simulink model "CSE1_CV3_1Straight"  (Simulink 7.3)
settings: Solver=ode4  StartTime=0.0  StopTime=inf  FixedStep=0.1  RelTol=1e-3
undefined symbols (not defined in the file or in its folder): eta1_0_real, v1_0_real, velocitySatValues1
libraries: simulink x68, dspmtrx3 x24, simulink_extras x23, marine_gnc x5, dspindex x5, dspinverses x4
(part 1 of 6)
settings Model: Creator=Dinh  LastModifiedBy=mcl  BufferReuse=off
settings DataIOCC: LimitDataPoints=off  SaveOutput=off  SaveTime=off
settings OptimizationCC: BlockReduction=off  BooleanDataType=off  ConditionallyExecuteInputs=off  OptimizeBlockIOStorage=off  BufferReuse=off  ExpressionFolding=off  LocalBlockOutputs=off  SimCompilerOptimization=On
settings DebuggingCC: InheritedTsInSrcMsg=none
settings SFSimCC: SimBuildMode=sf_nonincremental_build
settings RTWCC: SystemTargetFile=nidll.tlc  TemplateMakefile=nidll_vc.tmf  Description=NI Real-Time Target for Release 2007b or later  ProcessScript=nidll_make_rtw_hook
settings STFCustomTargetCC: MatFileLogging=on  SystemTargetFile=nidll.tlc

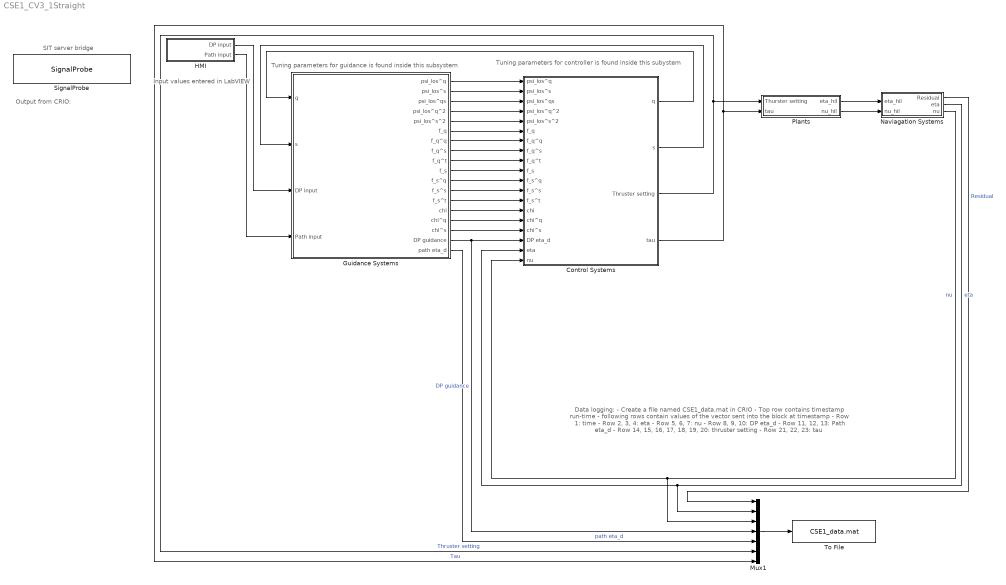
== system CSE1_CV3_1Straight ==
  note: Output from CRIO:
  note: SIT server bridge
  note: Tuning parameters for controller is found inside this subystem
  note: Tuning parameters for guidance is found inside this subsystem
  note: Input values entered
      |  in LabVIEW
  note: Data logging:
      | - Create a file named CSE1_data.mat in CRIO
      | - Top row contains timestamp run-time
      | - following rows contain values of the vector sent into the block at timestamp
      | - Row 1: time
      | - Row 2, 3, 4: eta
      | - Row 5, 6, 7: nu
      | - Row 8, 9, 10: DP eta_d
      | - Row 11, 12, 13: Path eta_d
      | - Row 14, 15, 16, 17, 18, 19, 20: thruster setting
      | - Row 21, 22, 23: tau
  Control Systems : Subsystem
  Guidance Systems : Subsystem
  HMI : Subsystem
  Mux1 : Mux  Inputs=7
  Naviagation Systems : Subsystem
      settings: MinAlgLoopOccurrences=on
  Plants : Subsystem
  SignalProbe : S-Function  Description=Use this block with SIT.  FunctionName=SignalProbe  Parameters=1  EnableBusSupport=off
      settings: PreSaveFcn=NISIT_ModelVars;
      mask Description: The LabVIEW Simulation Interface Toolkit uses the SignalProbe block to probe the signals in the model. The SignalProbe block must be on the top level of the model hierarchy. You can have only one SignalProbe block per model file. Do not rename the SignalProbe block. Do not change the name of another model block to SignalProbe.
  To File : ToFile  Filename=CSE1_data.mat  MatrixName=cse1_data
  wires:
  Control Systems/3(Thruster setting) -> Plants/1(Thurster setting), Mux1/6  "Thruster setting"
  Guidance Systems/17(DP guidance) -> Control Systems/17(DP eta_d), Mux1/4  "DP guidance"
  Plants/1(eta_hil) -> Naviagation Systems/1(eta_hil)
  Plants/2(nu_hil) -> Naviagation Systems/2(nu_hil)
  Naviagation Systems/2(eta) -> Mux1/2, Control Systems/18(eta)  "eta"
  Naviagation Systems/3(nu) -> Control Systems/19(nu), Mux1/3  "nu"
  Mux1/1 -> To File/1
  HMI/1(DP input) -> Guidance Systems/3(DP input)
  Control Systems/1(q) -> Guidance Systems/1(q)
  Control Systems/2(s) -> Guidance Systems/2(s)
  Control Systems/4(tau) -> Plants/2(tau), Mux1/7  "Tau"
  Naviagation Systems/1(Residual) -> Mux1/1  "Residual"
  HMI/2(Path input) -> Guidance Systems/4(Path input)
  Guidance Systems/18(path eta_d) -> Mux1/5  "path eta_d"
  Guidance Systems/1(psi_los^q) -> Control Systems/1(psi_los^q)
  Guidance Systems/2(psi_los^s) -> Control Systems/2(psi_los^s)
  Guidance Systems/3(psi_los^qs) -> Control Systems/3(psi_los^qs)
  Guidance Systems/4(psi_los^q^2) -> Control Systems/4(psi_los^q^2)
  Guidance Systems/5(psi_los^s^2) -> Control Systems/5(psi_los^s^2)
  Guidance Systems/6(f_q) -> Control Systems/6(f_q)
  Guidance Systems/7("f_q^q ") -> Control Systems/7(f_q^q)
  Guidance Systems/8(f_q^s) -> Control Systems/8(f_q^s)
  Guidance Systems/9(f_q^t) -> Control Systems/9(f_q^t)
  Guidance Systems/10(f_s) -> Control Systems/10(f_s)
  Guidance Systems/11(f_s^q) -> Control Systems/11(f_s^q)
  Guidance Systems/12(f_s^s) -> Control Systems/12(f_s^s)
  Guidance Systems/13(f_s^t) -> Control Systems/13(f_s^t)
  Guidance Systems/15(chi^q) -> Control Systems/15(chi^q)
  Guidance Systems/16(chi^s) -> Control Systems/16(chi^s)
  Guidance Systems/14(chi) -> Control Systems/14(chi)

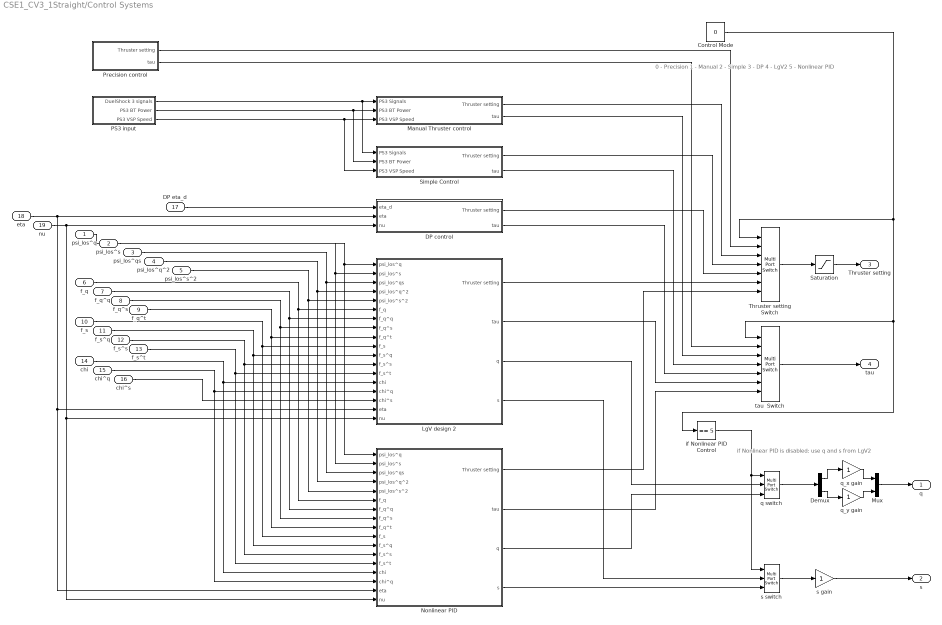
== system CSE1_CV3_1Straight/Control Systems ==
  note: 0 - Precision
      | 1 - Manual
      | 2 - Simple
      | 3 - DP
      | 4 - LgV2
      | 5 - Nonlinear PID
  note: if Nonlinear PID is disabled:
      |  use q and s from LgV2
  psi_los^q : Inport
  psi_los^s : Inport  Port=2
  psi_los^qs : Inport  Port=3
  psi_los^q^2 : Inport  Port=4
  psi_los^s^2 : Inport  Port=5
  f_q : Inport  Port=6
  f_q^q : Inport  Port=7
  f_q^s : Inport  Port=8
  f_q^t : Inport  Port=9
  f_s : Inport  Port=10
  f_s^q : Inport  Port=11
  f_s^s : Inport  Port=12
  f_s^t : Inport  Port=13
  chi : Inport  Port=14
  chi^q : Inport  Port=15
  chi^s : Inport  Port=16
  DP eta_d : Inport  Port=17
  eta : Inport  Port=18
  nu : Inport  Port=19
  Control Mode : Constant  Value=0
  DP control : Subsystem
  Demux : Demux  Outputs=2
  LgV design 2 : Subsystem
  Manual Thruster control : Subsystem
      settings: MinAlgLoopOccurrences=on
  Mux : Mux  Inputs=2
  Nonlinear PID : Subsystem
  PS3 input : Subsystem
  Precision control : Subsystem
  Saturation : Saturate  UpperLimit=1.0  LowerLimit=-1.0
  Simple Control : Subsystem
      settings: MinAlgLoopOccurrences=on
  Thruster setting Switch : MultiPortSwitch  Inputs=6  zeroidx=on
  if Nonlinear PID Control : simulink/Logic and Bit Operations/Compare To Constant  SystemSampleTime=-1  relop===  const=5  LogicOutDataTypeMode=uint8
  q switch : MultiPortSwitch  Inputs=2  zeroidx=on
  q_x gain : Gain  ParameterDataType=fixdt(1, 16)  ParameterScaling=2^0  OutDataType=fixdt(1, 16)  OutScaling=2^0
  q_y gain : Gain  ParameterDataType=fixdt(1, 16)  ParameterScaling=2^0  OutDataType=fixdt(1, 16)  OutScaling=2^0
  s gain : Gain  ParameterDataType=fixdt(1, 16)  ParameterScaling=2^0  OutDataType=fixdt(1, 16)  OutScaling=2^0
  s switch : MultiPortSwitch  Inputs=2  zeroidx=on
  tau  Switch : MultiPortSwitch  Inputs=6  zeroidx=on
  q : Outport
  s : Outport  Port=2
  Thruster setting : Outport  Port=3  PortDimensions=7
  tau : Outport  Port=4
  wires:
  DP eta_d/1 -> DP control/1(eta_d)
  nu/1 -> DP control/3(nu), LgV design 2/18(nu), Nonlinear PID/17(nu)
  eta/1 -> DP control/2(eta), LgV design 2/17(eta), Nonlinear PID/16(eta)
  Control Mode/1 -> Thruster setting Switch/1, tau  Switch/1, if Nonlinear PID Control/1
  Thruster setting Switch/1 -> Saturation/1
  Saturation/1 -> Thruster setting/1
  PS3 input/1(DuelShock 3 signals) -> Manual Thruster control/1(PS3 Signals), Simple Control/1(PS3 Signals)
  PS3 input/2(PS3 BT Power) -> Manual Thruster control/2(PS3 BT Power), Simple Control/2(PS3 BT Power)
  PS3 input/3(PS3 VSP Speed) -> Manual Thruster control/3(PS3 VSP Speed), Simple Control/3(PS3 VSP Speed)
  q switch/1 -> Demux/1
  s switch/1 -> s gain/1
  tau  Switch/1 -> tau/1
  Precision control/1(Thruster setting) -> Thruster setting Switch/2
  Nonlinear PID/4(s) -> s switch/3
  Manual Thruster control/1(Thruster setting) -> Thruster setting Switch/3
  Simple Control/1(Thruster setting) -> Thruster setting Switch/4
  DP control/1(Thruster setting) -> Thruster setting Switch/5
  LgV design 2/1(Thruster setting) -> Thruster setting Switch/6
  Precision control/2(tau) -> tau  Switch/2
  Manual Thruster control/2(tau) -> tau  Switch/3
  Simple Control/2(tau) -> tau  Switch/4
  DP control/2(tau) -> tau  Switch/5
  LgV design 2/2(tau) -> tau  Switch/6
  Nonlinear PID/1(Thruster setting) -> Thruster setting Switch/7
  Nonlinear PID/2(tau) -> tau  Switch/7
  LgV design 2/3(q) -> q switch/2
  Nonlinear PID/3(q) -> q switch/3
  if Nonlinear PID Control/1 -> s switch/1, q switch/1
  psi_los^q/1 -> LgV design 2/1(psi_los^q), Nonlinear PID/1(psi_los^q)
  psi_los^s/1 -> LgV design 2/2(psi_los^s), Nonlinear PID/2(psi_los^s)
  psi_los^qs/1 -> LgV design 2/3(psi_los^qs), Nonlinear PID/3(psi_los^qs)
  psi_los^q^2/1 -> LgV design 2/4(psi_los^q^2), Nonlinear PID/4(psi_los^q^2)
  psi_los^s^2/1 -> LgV design 2/5(psi_los^s^2), Nonlinear PID/5(psi_los^s^2)
  f_q/1 -> LgV design 2/6(f_q), Nonlinear PID/6(f_q)
  f_q^q/1 -> LgV design 2/7(f_q^q), Nonlinear PID/7(f_q^q)
  f_q^s/1 -> LgV design 2/8(f_q^s), Nonlinear PID/8(f_q^s)
  f_q^t/1 -> LgV design 2/9(f_q^t), Nonlinear PID/9(f_q^t)
  f_s/1 -> LgV design 2/10(f_s), Nonlinear PID/10(f_s)
  f_s^q/1 -> LgV design 2/11(f_s^q), Nonlinear PID/11(f_s^q)
  f_s^s/1 -> LgV design 2/12(f_s^s), Nonlinear PID/12(f_s^s)
  f_s^t/1 -> LgV design 2/13(f_s^t), Nonlinear PID/13(f_s^t)
  chi/1 -> LgV design 2/14(chi), Nonlinear PID/14(chi)
  chi^q/1 -> LgV design 2/15(chi^q), Nonlinear PID/15(chi^q)
  chi^s/1 -> LgV design 2/16(chi^s)
  s gain/1 -> s/1
  Demux/1 -> q_x gain/1
  Demux/2 -> q_y gain/1
  q_x gain/1 -> Mux/1
  q_y gain/1 -> Mux/2
  Mux/1 -> q/1
  LgV design 2/4(s) -> s switch/2

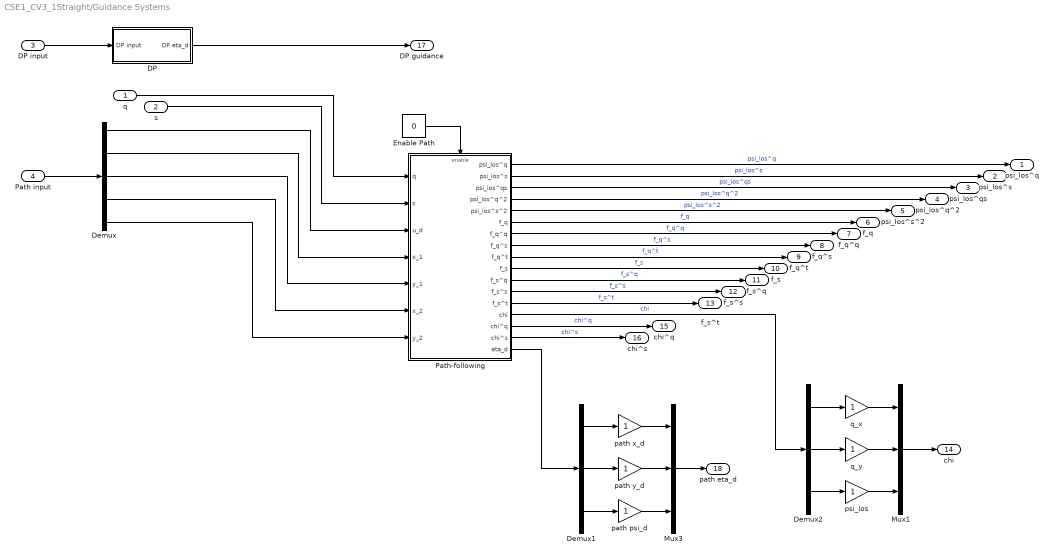
== system CSE1_CV3_1Straight/Guidance Systems ==
  q : Inport
  s : Inport  Port=2
  DP input : Inport  Port=3
  Path input : Inport  Port=4
  DP : Subsystem
  Demux : Demux  Outputs=5
  Demux1 : Demux  Outputs=3
  Demux2 : Demux  Outputs=3
  Enable Path : Constant  Value=0
  Mux1 : Mux  Inputs=3
  Mux3 : Mux  Inputs=3
  Path-following : Subsystem
  path psi_d : Gain  ParameterDataType=fixdt(1, 16)  ParameterScaling=2^0  OutDataType=fixdt(1, 16)  OutScaling=2^0
  path x_d : Gain  ParameterDataType=fixdt(1, 16)  ParameterScaling=2^0  OutDataType=fixdt(1, 16)  OutScaling=2^0
  path y_d : Gain  ParameterDataType=fixdt(1, 16)  ParameterScaling=2^0  OutDataType=fixdt(1, 16)  OutScaling=2^0
  psi_los : Gain  ParameterDataType=fixdt(1, 16)  ParameterScaling=2^0  OutDataType=fixdt(1, 16)  OutScaling=2^0
  q_x : Gain  ParameterDataType=fixdt(1, 16)  ParameterScaling=2^0  OutDataType=fixdt(1, 16)  OutScaling=2^0
  q_y : Gain  ParameterDataType=fixdt(1, 16)  ParameterScaling=2^0  OutDataType=fixdt(1, 16)  OutScaling=2^0
  psi_los^q : Outport
  psi_los^s : Outport  Port=2
  psi_los^qs : Outport  Port=3
  psi_los^q^2 : Outport  Port=4
  psi_los^s^2 : Outport  Port=5
  f_q : Outport  Port=6
  "f_q^q " : Outport  Port=7
  f_q^s : Outport  Port=8
  f_q^t : Outport  Port=9
  f_s : Outport  Port=10
  f_s^q : Outport  Port=11
  f_s^s : Outport  Port=12
  f_s^t : Outport  Port=13
  chi : Outport  Port=14
  chi^q : Outport  Port=15
  chi^s : Outport  Port=16
  DP guidance : Outport  Port=17
  path eta_d : Outport  Port=18
  wires:
  DP/1(DP eta_d) -> DP guidance/1
  DP input/1 -> DP/1(DP input)
  q/1 -> Path-following/1(q)
  s/1 -> Path-following/2(s)
  Demux/1 -> Path-following/3(u_d)
  Demux/2 -> Path-following/4(x_1)
  Demux/3 -> Path-following/5(y_1)
  Demux/4 -> Path-following/6(x_2)
  Path-following/1(psi_los^q) -> psi_los^q/1  "psi_los^q"
  Path-following/2(psi_los^s) -> psi_los^s/1  "psi_los^s"
  Path-following/3(psi_los^qs) -> psi_los^qs/1  "psi_los^qs"
  Path-following/4(psi_los^q^2) -> psi_los^q^2/1  "psi_los^q^2"
  Path-following/5(psi_los^s^2) -> psi_los^s^2/1  "psi_los^s^2"
  Path-following/6(f_q) -> f_q/1  "f_q"
  Path-following/7("f_q^q ") -> "f_q^q "/1  "f_q^q"
  Path-following/8(f_q^s) -> f_q^s/1  "f_q^s"
  Path-following/9(f_q^t) -> f_q^t/1  "f_q^t"
  Path-following/10(f_s) -> f_s/1  "f_s"
  Path-following/11(f_s^q) -> f_s^q/1  "f_s^q"
  Path-following/12(f_s^s) -> f_s^s/1  "f_s^s"
  Path-following/13(f_s^t) -> f_s^t/1  "f_s^t"
  Path-following/14(chi) -> Demux2/1  "chi"
  Path-following/15(chi^q) -> chi^q/1  "chi^q"
  Path-following/16(chi^s) -> chi^s/1  "chi^s"
  Path input/1 -> Demux/1
  Demux/5 -> Path-following/7(y_2)
  Demux1/1 -> path x_d/1
  Demux1/2 -> path y_d/1
  Demux1/3 -> path psi_d/1
  path x_d/1 -> Mux3/1
  path psi_d/1 -> Mux3/3
  path y_d/1 -> Mux3/2
  Mux3/1 -> path eta_d/1
  Path-following/17(eta_d) -> Demux1/1
  Demux2/1 -> q_x/1
  Demux2/2 -> q_y/1
  Demux2/3 -> psi_los/1
  q_x/1 -> Mux1/1
  psi_los/1 -> Mux1/3
  q_y/1 -> Mux1/2
  Mux1/1 -> chi/1
  Enable Path/1 -> Path-following/Enable

== system CSE1_CV3_1Straight/HMI ==
  DP Input : Subsystem
  Path-following input : Subsystem
  DP input : Outport
  Path input : Outport  Port=2
  wires:
  DP Input/1(DP input) -> DP input/1
  Path-following input/1(Path input) -> Path input/1

== system CSE1_CV3_1Straight/Naviagation Systems ==
  eta_hil : Inport
  nu_hil : Inport  Port=2
  Controller Input Selector : Constant  Value=0
  Demux : Demux  Outputs=3
  Demux1 : Demux  Outputs=3
  Eta Switch : MultiPortSwitch  Inputs=2  zeroidx=on
  Mux1 : Mux  Inputs=3
  Mux3 : Mux  Inputs=3
  Nu Switch : MultiPortSwitch  Inputs=2  zeroidx=on
  Qualisys 6 DOF : Subsystem
  eta_surge : Gain  ParameterDataType=fixdt(1, 16)  ParameterScaling=2^0  OutDataType=fixdt(1, 16)  OutScaling=2^0
  eta_sway : Gain  ParameterDataType=fixdt(1, 16)  ParameterScaling=2^0  OutDataType=fixdt(1, 16)  OutScaling=2^0
  eta_yaw : Gain  ParameterDataType=fixdt(1, 16)  ParameterScaling=2^0  OutDataType=fixdt(1, 16)  OutScaling=2^0
  nu_surge : Gain  ParameterDataType=fixdt(1, 16)  ParameterScaling=2^0  OutDataType=fixdt(1, 16)  OutScaling=2^0
  nu_sway : Gain  ParameterDataType=fixdt(1, 16)  ParameterScaling=2^0  OutDataType=fixdt(1, 16)  OutScaling=2^0
  nu_yaw : Gain  ParameterDataType=fixdt(1, 16)  ParameterScaling=2^0  OutDataType=fixdt(1, 16)  OutScaling=2^0
  Residual : Outport
  eta : Outport  Port=2
  nu : Outport  Port=3
  wires:
  Controller Input Selector/1 -> Eta Switch/1, Nu Switch/1
  Qualisys 6 DOF/1(eta_qs) -> Eta Switch/2
  Qualisys 6 DOF/2(nu_qs) -> Nu Switch/2
  eta_hil/1 -> Eta Switch/3
  nu_hil/1 -> Nu Switch/3
  Demux/1 -> eta_surge/1
  Demux/2 -> eta_sway/1
  Demux/3 -> eta_yaw/1
  eta_surge/1 -> Mux3/1
  eta_yaw/1 -> Mux3/3
  eta_sway/1 -> Mux3/2
  Mux3/1 -> eta/1
  Demux1/1 -> nu_surge/1
  Demux1/2 -> nu_sway/1
  Demux1/3 -> nu_yaw/1
  nu_surge/1 -> Mux1/1
  nu_sway/1 -> Mux1/2
  nu_yaw/1 -> Mux1/3
  Mux1/1 -> nu/1
  Nu Switch/1 -> Demux1/1
  Eta Switch/1 -> Demux/1
  Qualisys 6 DOF/3(Residual) -> Residual/1

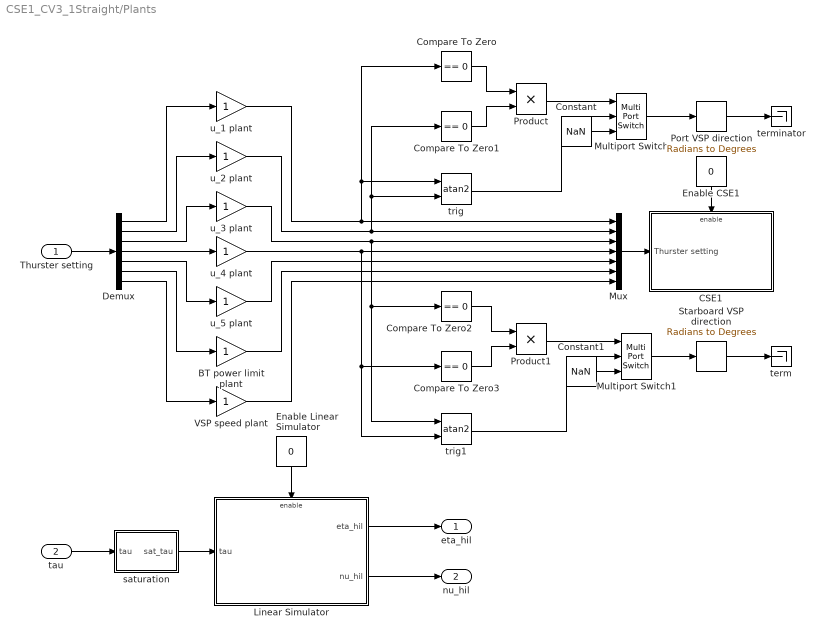
== system CSE1_CV3_1Straight/Plants ==
  Thurster setting : Inport
  tau : Inport  Port=2
  BT power limit plant : Gain  ParameterDataType=fixdt(1, 16)  ParameterScaling=2^0  OutDataType=fixdt(1, 16)  OutScaling=2^0
  CSE1 : Subsystem
  Compare To Zero{,1..3} (4 alike) : simulink/Logic and Bit Operations/Compare To Zero  SystemSampleTime=-1  relop===  LogicOutDataTypeMode=uint8  ZeroCross=off
  Constant : Constant  Value=NaN  OutDataType=fixdt(1, 16)  OutScaling=2^0
  Constant1 : Constant  Value=NaN  OutDataType=fixdt(1, 16)  OutScaling=2^0
  Demux : Demux  Outputs=7
  Enable CSE1 : Constant  Value=0
  Enable Linear Simulator : Constant  Value=0
  Linear Simulator : Subsystem
      settings: MinAlgLoopOccurrences=on
  Multiport Switch : MultiPortSwitch  Inputs=2  zeroidx=on  OutDataType=fixdt(1, 16)  OutScaling=2^0
  Multiport Switch1 : MultiPortSwitch  Inputs=2  zeroidx=on  OutDataType=fixdt(1, 16)  OutScaling=2^0
  Mux : Mux  Inputs=7
  Port VSP direction : simulink_extras/Transformations/Radians to Degrees  SystemSampleTime=-1
  Product : Product  OutDataType=fixdt(1, 16)  OutScaling=2^0  RndMeth=Zero
  Product1 : Product  OutDataType=fixdt(1, 16)  OutScaling=2^0  RndMeth=Zero
  Starboard VSP direction : simulink_extras/Transformations/Radians to Degrees  SystemSampleTime=-1
  VSP speed plant : Gain  ParameterDataType=fixdt(1, 16)  ParameterScaling=2^0  OutDataType=fixdt(1, 16)  OutScaling=2^0
  saturation : Subsystem  AncestorBlock=marine_gnc/Examples/Vessels/CyberShipII/saturation
  term : Terminator
  terminator : Terminator
  trig : Trigonometry  Operator=atan2
  trig1 : Trigonometry  Operator=atan2
  u_1 plant : Gain  ParameterDataType=fixdt(1, 16)  ParameterScaling=2^0  OutDataType=fixdt(1, 16)  OutScaling=2^0
  u_2 plant : Gain  ParameterDataType=fixdt(1, 16)  ParameterScaling=2^0  OutDataType=fixdt(1, 16)  OutScaling=2^0
  u_3 plant : Gain  ParameterDataType=fixdt(1, 16)  ParameterScaling=2^0  OutDataType=fixdt(1, 16)  OutScaling=2^0
  u_4 plant : Gain  ParameterDataType=fixdt(1, 16)  ParameterScaling=2^0  OutDataType=fixdt(1, 16)  OutScaling=2^0
  u_5 plant : Gain  ParameterDataType=fixdt(1, 16)  ParameterScaling=2^0  OutDataType=fixdt(1, 16)  OutScaling=2^0
  eta_hil : Outport
  nu_hil : Outport  Port=2
  wires:
  Linear Simulator/1(eta_hil) -> eta_hil/1
  Linear Simulator/2(nu_hil) -> nu_hil/1
  Enable CSE1/1 -> CSE1/Enable
  Enable Linear Simulator/1 -> Linear Simulator/Enable
  Thurster setting/1 -> Demux/1
  Mux/1 -> CSE1/1(Thurster setting)
  Demux/1 -> u_1 plant/1
  Demux/2 -> u_2 plant/1
  Demux/3 -> u_3 plant/1
  Demux/4 -> u_4 plant/1
  u_4 plant/1 -> Mux/4, trig1/2, Compare To Zero3/1
  u_1 plant/1 -> Mux/1, trig/1, Compare To Zero/1
  u_2 plant/1 -> Mux/2, trig/2, Compare To Zero1/1
  u_3 plant/1 -> Mux/3, trig1/1, Compare To Zero2/1
  Demux/5 -> u_5 plant/1
  Demux/6 -> BT power limit plant/1
  Demux/7 -> VSP speed plant/1
  u_5 plant/1 -> Mux/5
  BT power limit plant/1 -> Mux/6
  VSP speed plant/1 -> Mux/7
  tau/1 -> saturation/1(tau)
  saturation/1(sat_tau) -> Linear Simulator/1(tau)
  Compare To Zero/1 -> Product/1
  Compare To Zero1/1 -> Product/2
  Product/1 -> Multiport Switch/1
  Multiport Switch/1 -> Port VSP direction/1
  trig/1 -> Multiport Switch/2
  Constant/1 -> Multiport Switch/3
  Compare To Zero2/1 -> Product1/1
  Compare To Zero3/1 -> Product1/2
  Product1/1 -> Multiport Switch1/1
  Multiport Switch1/1 -> Starboard VSP direction/1
  trig1/1 -> Multiport Switch1/2
  Constant1/1 -> Multiport Switch1/3
  Port VSP direction/1 -> terminator/1
  Starboard VSP direction/1 -> term/1

== system CSE1_CV3_1Straight/Control Systems/DP control ==
  eta_d : Inport
  eta : Inport  Port=2
  nu : Inport  Port=3
  BT_power_limit : Constant  Value=0.5
  DP controller : Subsystem  mask(Nonlinear DP Controller){Kp=(0.1)^2*[25.8000 0  0;  0  33.8000  1.0115;  0  1.0115  2.7600 ], Kd=2*0.8*0.1*[25.8000 0  0;  0  33.8000  1.0115;  0  1.0115  2.7600 ], Ki=(0.1^3/10)*[25.8000 0  0;  0  33.8000  1.0115;  0  1.0115  2.7600 ]}
      mask prompts: Kp "Proportional Gain Matrix: Kp"; Kd "Derivative Gain Matrix: Kd"; Ki "Integral Gain Matrix: Ki"
      mask help: Nonlinear PID controller for Set-Point Reulation in Surge, Sway and Yaw
      mask Help:
      | The nonlinear  PID controller uses the rotation matrix in yaw for proper scaling of the surge, sway and yaw gains as a function of the yaw angle.
      | INPUTS: (1) eta_ref, (2) eta, (3) nu. OUPUTS: (1) tau.
      mask Display: disp('Nonlinear PID\n set-point controller')
  DP tau_surge : Gain  ParameterDataType=fixdt(1, 16)  ParameterScaling=2^0  OutDataType=fixdt(1, 16)  OutScaling=2^0
  DP tau_sway : Gain  ParameterDataType=fixdt(1, 16)  ParameterScaling=2^0  OutDataType=fixdt(1, 16)  OutScaling=2^0
  DP tau_yaw : Gain  ParameterDataType=fixdt(1, 16)  ParameterScaling=2^0  OutDataType=fixdt(1, 16)  OutScaling=2^0
  DP u_{1..5} (5 alike) : Gain  ParameterDataType=fixdt(1, 16)  ParameterScaling=2^0  OutDataType=fixdt(1, 16)  OutScaling=2^0
  Demux : Demux  Outputs=3
  Demux1 : Demux  Outputs=5
  Enable Filter : Constant  Value=0
  Multiport Switch : MultiPortSwitch  Inputs=2  zeroidx=on
  Multiport Switch1 : MultiPortSwitch  Inputs=2  zeroidx=on
  Mux1 : Mux  Inputs=3
  Mux2 : Mux  Inputs=5
  Mux3 : Mux  Inputs=3
  Passive DP wave filter1 : marine_gnc/Navigation/Observers/Passive DP wave filter  SystemSampleTime=-1  lambda=0.1*diag([1 1 1])  w_o=diag([0.8 0.8 0.8])  K4=0.1*diag([1 1 0.1])  K3=0.1*diag([1 1 0.1])  w_c=1.3*diag([0.8 0.8 0.8])  T_b=diag([100 100 100])  M="[ 25.8000   0    0;   0   33.8000   1.0115; 0   1.0115    2.7600 ]"  D="[2 0  0;  0 7 0.1; 0 0.1 0.5]"
  Saturation : Saturate  UpperLimit=1.0  LowerLimit=-1.0
  Thruster allocation : Subsystem
  To File : ToFile  Filename=CSE1_data_eta_w.mat  MatrixName=cse1_data
  VSP_speeds : Constant  Value=0.4
  Thruster setting : Outport  InitialOutput=[0;0;0;0;0;0;0]
  tau : Outport  Port=2
  wires:
  Mux1/1 -> Thruster setting/1
  eta_d/1 -> DP controller/1(eta_ref)
  eta/1 -> Passive DP wave filter1/1, Multiport Switch/2
  nu/1 -> Multiport Switch1/2
  Multiport Switch/1 -> DP controller/2(eta)
  Multiport Switch1/1 -> DP controller/3(nu)
  Passive DP wave filter1/2 -> Multiport Switch/3
  Passive DP wave filter1/3 -> Multiport Switch1/3
  Enable Filter/1 -> Multiport Switch/1, Multiport Switch1/1
  Saturation/1 -> Mux1/1
  Passive DP wave filter1/1 -> To File/1
  BT_power_limit/1 -> Mux1/2
  VSP_speeds/1 -> Mux1/3
  Demux/1 -> DP tau_surge/1
  Demux/2 -> DP tau_sway/1
  Demux/3 -> DP tau_yaw/1
  DP tau_surge/1 -> Mux3/1
  DP tau_yaw/1 -> Mux3/3
  DP tau_sway/1 -> Mux3/2
  DP controller/1(tau) -> Demux/1
  Mux3/1 -> Thruster allocation/1(tau), Passive DP wave filter1/2, tau/1
  Demux1/1 -> DP u_1/1
  Demux1/2 -> DP u_2/1
  Demux1/3 -> DP u_3/1
  DP u_1/1 -> Mux2/1
  DP u_3/1 -> Mux2/3
  DP u_2/1 -> Mux2/2
  Demux1/4 -> DP u_4/1
  Demux1/5 -> DP u_5/1
  DP u_4/1 -> Mux2/4
  DP u_5/1 -> Mux2/5
  Mux2/1 -> Saturation/1
  Thruster allocation/1(u_act) -> Demux1/1

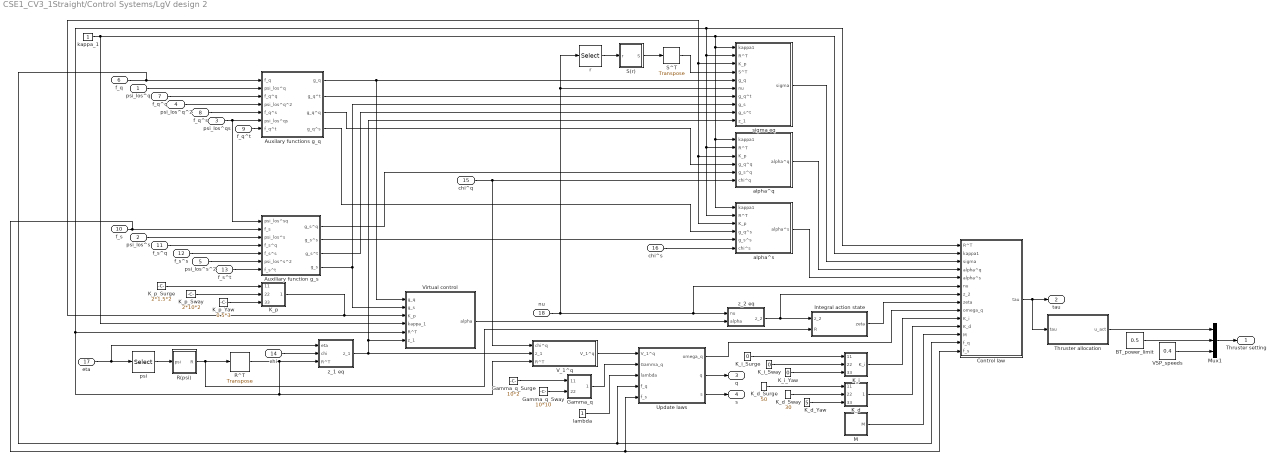
== system CSE1_CV3_1Straight/Control Systems/LgV design 2 ==
  psi_los^q : Inport
  psi_los^s : Inport  Port=2
  psi_los^qs : Inport  Port=3
  psi_los^q^2 : Inport  Port=4
  psi_los^s^2 : Inport  Port=5
  f_q : Inport  Port=6
  f_q^q : Inport  Port=7
  f_q^s : Inport  Port=8
  f_q^t : Inport  Port=9
  f_s : Inport  Port=10
  f_s^q : Inport  Port=11
  f_s^s : Inport  Port=12
  f_s^t : Inport  Port=13
  chi : Inport  Port=14
  chi^q : Inport  Port=15
  chi^s : Inport  Port=16
  eta : Inport  Port=17
  nu : Inport  Port=18
  Auxilary functions g_q : Subsystem
  Auxiliary function g_s : Subsystem
  BT_power_limit : Constant  Value=0.5
  Control law : Subsystem
  Gamma_q : Subsystem
  Gamma_q_Surge : Constant  Value=10*2
  Gamma_q_Sway : Constant  Value=10*10
  Integral action state : Subsystem
  K_d : Subsystem
  K_d_Surge : Constant  Value=50
  K_d_Sway : Constant  Value=30
  K_d_Yaw : Constant  Value=5
  K_i : Subsystem
  K_i_Surge : Constant  Value=0
  K_i_Sway : Constant  Value=0
  K_i_Yaw : Constant  Value=0
  K_p : Subsystem
  K_p_Surge : Constant  Value=2*1.5*2
  K_p_Sway : Constant  Value=2*10*2
  K_p_Yaw : Constant  Value=0.5*3
  M : Subsystem
  Mux1 : Mux  Inputs=3
  R(psi) : Subsystem
  R^T : dspmtrx3/Transpose  SystemSampleTime=-1  Hermitian=off  overflowFlag=off
  S(r) : Subsystem
  S^T : dspmtrx3/Transpose  SystemSampleTime=-1  Hermitian=off  overflowFlag=off
  Thruster allocation : Subsystem
  Update laws : Subsystem
  VSP_speeds : Constant  Value=0.4
  V_1^q : Subsystem
  Virtual control : Subsystem
  alpha^q : Subsystem
  alpha^s : Subsystem
  kappa_1 : Constant
  lambda : Constant
  psi : Selector  InputPortWidth=3  IndexOptions=Index vector (dialog)  Indices=[3]  OutputSizes=1
  r : Selector  InputPortWidth=3  IndexOptions=Index vector (dialog)  Indices=[3]  OutputSizes=1
  sigma eq : Subsystem
  z_1 eq : Subsystem
  z_2 eq : Subsystem
  Thruster setting : Outport  InitialOutput=[0;0;0;0;0;0;0]
  tau : Outport  Port=2
  q : Outport  Port=3
  s : Outport  Port=4
  wires:
  psi/1 -> R(psi)/1(psi)
  eta/1 -> psi/1, z_1 eq/1(eta)
  R(psi)/1(R) -> R^T/1, Integral action state/2(R)
  nu/1 -> z_2 eq/1(nu), Control law/6(nu), r/1, sigma eq/6(nu)
  Virtual control/1(alpha) -> z_2 eq/2(alpha)
  psi_los^q/1 -> Auxilary functions g_q/2(psi_los^q)
  K_p/1(K_p) -> Virtual control/3(K_p), sigma eq/3(K_p), alpha^q/3(K_p), alpha^s/3(K_p)
  kappa_1/1 -> Virtual control/4(kappa_1), Control law/2(kappa1), sigma eq/1(kappa1), alpha^q/1(kappa1), alpha^s/1(kappa1)
  Control law/1(tau) -> tau/1, Thruster allocation/1(tau)
  z_1 eq/1(z_1) -> V_1^q/2(z_1), Virtual control/6(z_1), sigma eq/10(z_1)
  R^T/1 -> z_1 eq/3(R^T), Virtual control/5(R^T), Control law/1(R^T), sigma eq/2(R^T), alpha^q/2(R^T), alpha^s/2(R^T), V_1^q/3(R^T)
  chi/1 -> z_1 eq/2(chi)
  K_p_Surge/1 -> K_p/1(11)
  K_p_Sway/1 -> K_p/2(22)
  K_p_Yaw/1 -> K_p/3(33)
  Update laws/1(omega_q) -> Control law/9(omega_q)
  V_1^q/1(V_1^q) -> Update laws/1(V_1^q)
  Update laws/2(q) -> q/1
  Update laws/3(s) -> s/1
  r/1 -> S(r)/1(r)
  S(r)/1(S) -> S^T/1
  f_s/1 -> Auxiliary function g_s/2(f_s), Update laws/5(f_s), Control law/14(f_s)
  psi_los^s/1 -> Auxiliary function g_s/3(psi_los^s)
  Auxilary functions g_q/1(g_q) -> sigma eq/5(g_q), Virtual control/1(g_q)
  Auxiliary function g_s/4(g_s) -> Virtual control/2(g_s), sigma eq/8(g_s)
  f_s^q/1 -> Auxiliary function g_s/4(f_s^q)
  f_s^s/1 -> Auxiliary function g_s/5(f_s^s)
  psi_los^s^2/1 -> Auxiliary function g_s/6(psi_los^s^2)
  f_s^t/1 -> Auxiliary function g_s/7(f_s^t)
  f_q^q/1 -> Auxilary functions g_q/3(f_q^q)
  psi_los^q^2/1 -> Auxilary functions g_q/4(psi_los^q^2)
  f_q^s/1 -> Auxilary functions g_q/5(f_q^s)
  psi_los^qs/1 -> Auxilary functions g_q/6(psi_los^qs), Auxiliary function g_s/1(psi_los^sq)
  f_q^t/1 -> Auxilary functions g_q/7(f_q^t)
  sigma eq/1(sigma) -> Control law/3(sigma)
  z_2 eq/1(z_2) -> Integral action state/1(z_2), Control law/7(z_2)
  lambda/1 -> Update laws/3(lambda)
  M/1(M) -> Control law/12(M)
  K_i_Surge/1 -> K_i/1(11)
  K_i_Sway/1 -> K_i/2(22)
  K_i_Yaw/1 -> K_i/3(33)
  K_d_Surge/1 -> K_d/1(11)
  K_d_Sway/1 -> K_d/2(22)
  K_d_Yaw/1 -> K_d/3(33)
  K_i/1(K_i) -> Control law/10(K_i)
  K_d/1(K_d) -> Control law/11(K_d)
  S^T/1 -> sigma eq/4(S^T)
  Auxiliary function g_s/3(g_s^t) -> sigma eq/9(g_s^t)
  Auxilary functions g_q/2(g_q^t) -> sigma eq/7(g_q^t)
  f_q/1 -> Auxilary functions g_q/1(f_q), Update laws/4(f_q), Control law/13(f_q)
  alpha^q/1(alpha^q) -> Control law/4(alpha^q)
  Auxilary functions g_q/3(g_q^q) -> alpha^q/4(g_q^q)
  Auxiliary function g_s/1(g_s^q) -> alpha^q/5(g_s^q)
  alpha^s/1(alpha^s) -> Control law/5(alpha^s)
  Auxiliary function g_s/2(g_s^s) -> alpha^s/5(g_s^s)
  chi^s/1 -> alpha^s/6(chi^s)
  Auxilary functions g_q/4(g_q^s) -> alpha^s/4(g_q^s)
  chi^q/1 -> alpha^q/6(chi^q), V_1^q/1(chi^q)
  Integral action state/1(zeta) -> Control law/8(zeta)
  Gamma_q/1(Gamma_q) -> Update laws/2(Gamma_q)
  Gamma_q_Surge/1 -> Gamma_q/1(11)
  Gamma_q_Sway/1 -> Gamma_q/2(22)
  Mux1/1 -> Thruster setting/1
  BT_power_limit/1 -> Mux1/2
  VSP_speeds/1 -> Mux1/3
  Thruster allocation/1(u_act) -> Mux1/1

== system CSE1_CV3_1Straight/Control Systems/Manual Thruster control ==
  note: Manuel thruster control is intended for testing and flexing of thrusters and its signals
  PS3 Signals : Inport
  PS3 BT Power : Inport  Port=2
  PS3 VSP Speed : Inport  Port=3
  Add : Sum  Inputs=|++
  Demux : Demux  Outputs=6
  Mux : Mux  Inputs=7
  PS3 u_{1..5} (5 alike) : Gain  ParameterDataType=fixdt(1, 16)  ParameterScaling=2^0  OutDataType=fixdt(1, 16)  OutScaling=2^0
  Subsystem : Subsystem
  Thruster setting : Outport
  tau : Outport  Port=2
  wires:
  PS3 Signals/1 -> Demux/1
  Demux/1 -> PS3 u_2/1  "Left/Right position of Left Joystick"
  Demux/2 -> PS3 u_1/1  "Up/Down position of Left Joystick"
  Demux/3 -> PS3 u_4/1  "Left/Right position of Right Joystick"
  Demux/4 -> PS3 u_3/1  "Up/Down position of Right Joystick"
  Demux/5 -> Add/1  "L2 signal"
  Demux/6 -> Add/2  "R2 signal"
  PS3 VSP Speed/1 -> Mux/7  "VPS Speed"
  PS3 BT Power/1 -> Mux/6  "Bow Thruster Limit"
  Add/1 -> PS3 u_5/1  "Bow Thruster direction"
  Mux/1 -> Thruster setting/1, Subsystem/1(u_act)
  PS3 u_1/1 -> Mux/1  "u_1"
  PS3 u_2/1 -> Mux/2  "u_2"
  PS3 u_5/1 -> Mux/5  "u_5"
  PS3 u_4/1 -> Mux/4  "u_4"
  PS3 u_3/1 -> Mux/3  "u_3"
  Subsystem/1(tau) -> tau/1

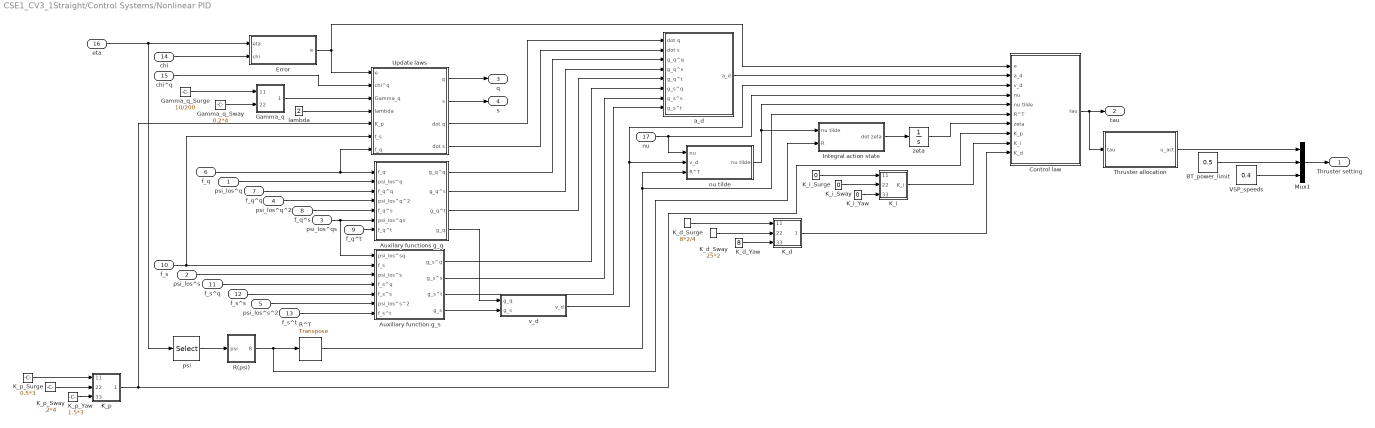
== system CSE1_CV3_1Straight/Control Systems/Nonlinear PID ==
  psi_los^q : Inport
  psi_los^s : Inport  Port=2
  psi_los^qs : Inport  Port=3
  psi_los^q^2 : Inport  Port=4
  psi_los^s^2 : Inport  Port=5
  f_q : Inport  Port=6
  f_q^q : Inport  Port=7
  f_q^s : Inport  Port=8
  f_q^t : Inport  Port=9
  f_s : Inport  Port=10
  f_s^q : Inport  Port=11
  f_s^s : Inport  Port=12
  f_s^t : Inport  Port=13
  chi : Inport  Port=14
  chi^q : Inport  Port=15
  eta : Inport  Port=16
  nu : Inport  Port=17
  Auxilary functions g_q : Subsystem
  Auxiliary function g_s : Subsystem
  BT_power_limit : Constant  Value=0.5
  Control law : Subsystem
  Error : Subsystem
  Gamma_q : Subsystem
  Gamma_q_Surge : Constant  Value=10/200
  Gamma_q_Sway : Constant  Value=0.2*4
  Integral action state : Subsystem
  K_d : Subsystem
  K_d_Surge : Constant  Value=8*2/4
  K_d_Sway : Constant  Value=25*2
  K_d_Yaw : Constant  Value=8
  K_i : Subsystem
  K_i_Surge : Constant  Value=0
  K_i_Sway : Constant  Value=0
  K_i_Yaw : Constant  Value=0
  K_p : Subsystem
  K_p_Surge : Constant  Value=0.5*3
  K_p_Sway : Constant  Value=.2*4
  K_p_Yaw : Constant  Value=1.5*3
  Mux1 : Mux  Inputs=3
  R(psi) : Subsystem
  R^T : dspmtrx3/Transpose  SystemSampleTime=-1  Hermitian=off  overflowFlag=off
  Thruster allocation : Subsystem
  Update laws : Subsystem
  VSP_speeds : Constant  Value=0.4
  a_d : Subsystem
  lambda : Constant  Value=2
  nu tilde : Subsystem
  psi : Selector  InputPortWidth=3  IndexOptions=Index vector (dialog)  Indices=[3]  OutputSizes=1
  v_d : Subsystem
  zeta : Integrator
  Thruster setting : Outport  InitialOutput=[0;0;0;0;0;0;0]
  tau : Outport  Port=2
  q : Outport  Port=3
  s : Outport  Port=4
  wires:
  psi/1 -> R(psi)/1(psi)
  R(psi)/1(R) -> R^T/1, Integral action state/2(R)
  psi_los^q/1 -> Auxilary functions g_q/2(psi_los^q)
  Control law/1(tau) -> tau/1, Thruster allocation/1(tau)
  Integral action state/1(dot zeta) -> zeta/1
  Update laws/1(q) -> q/1
  f_s/1 -> Auxiliary function g_s/2(f_s), Update laws/6(f_s)
  psi_los^s/1 -> Auxiliary function g_s/3(psi_los^s)
  f_s^q/1 -> Auxiliary function g_s/4(f_s^q)
  f_s^s/1 -> Auxiliary function g_s/5(f_s^s)
  psi_los^s^2/1 -> Auxiliary function g_s/6(psi_los^s^2)
  f_s^t/1 -> Auxiliary function g_s/7(f_s^t)
  f_q^q/1 -> Auxilary functions g_q/3(f_q^q)
  psi_los^q^2/1 -> Auxilary functions g_q/4(psi_los^q^2)
  f_q^s/1 -> Auxilary functions g_q/5(f_q^s)
  psi_los^qs/1 -> Auxilary functions g_q/6(psi_los^qs), Auxiliary function g_s/1(psi_los^sq)
  f_q^t/1 -> Auxilary functions g_q/7(f_q^t)
  lambda/1 -> Update laws/4(lambda)
  K_d_Surge/1 -> K_d/1(11)
  K_i/1(K_i) -> Control law/9(K_i)
  K_d/1(K_d) -> Control law/10(K_d)
  f_q/1 -> Auxilary functions g_q/1(f_q), Update laws/7(f_q)
  chi^q/1 -> Update laws/2(chi^q)
  K_p/1(K_p) -> Control law/8(K_p), Update laws/5(K_p)
  nu/1 -> Control law/4(nu), nu tilde/1(nu)
  Error/1(e) -> Update laws/1(e), Control law/1(e)
  v_d/1(v_d) -> Control law/3(v_d), nu tilde/2(v_d)
  Update laws/3(dot q) -> a_d/1(dot q)
  Update laws/4(dot s) -> a_d/2(dot s)
  Auxiliary function g_s/4(g_s) -> v_d/2(g_s)
  Auxilary functions g_q/4(g_q) -> v_d/1(g_q)
  Auxilary functions g_q/1(g_q^q) -> a_d/3(g_q^q)
  Auxilary functions g_q/2(g_q^s) -> a_d/4(g_q^s)
  Auxilary functions g_q/3(g_q^t) -> a_d/5(g_q^t)
  Auxiliary function g_s/1(g_s^q) -> a_d/6(g_s^q)
  Auxiliary function g_s/2(g_s^s) -> a_d/7(g_s^s)
  Auxiliary function g_s/3(g_s^t) -> a_d/8(g_s^t)
  chi/1 -> Error/2(chi)
  eta/1 -> psi/1, Error/1(eta)
  R^T/1 -> nu tilde/3(R^T), Control law/6(R^T)
  a_d/1(a_d) -> Control law/2(a_d)
  zeta/1 -> Control law/7(zeta)
  nu tilde/1(nu tilde) -> Control law/5(nu tilde), Integral action state/1(nu tilde)
  K_p_Surge/1 -> K_p/1(11)
  K_p_Sway/1 -> K_p/2(22)
  K_p_Yaw/1 -> K_p/3(33)
  K_d_Sway/1 -> K_d/2(22)
  K_d_Yaw/1 -> K_d/3(33)
  K_i_Surge/1 -> K_i/1(11)
  K_i_Sway/1 -> K_i/2(22)
  K_i_Yaw/1 -> K_i/3(33)
  Gamma_q_Surge/1 -> Gamma_q/1(11)
  Gamma_q_Sway/1 -> Gamma_q/2(22)
  Gamma_q/1(Gamma_q) -> Update laws/3(Gamma_q)
  Mux1/1 -> Thruster setting/1
  BT_power_limit/1 -> Mux1/2
  VSP_speeds/1 -> Mux1/3
  Thruster allocation/1(u_act) -> Mux1/1
  Update laws/2(s) -> s/1

== system CSE1_CV3_1Straight/Control Systems/PS3 input ==
  AS_LX : Constant  Value=0
  AS_LY : Constant  Value=0
  AS_RX : Constant  Value=0
  AS_RY : Constant  Value=0
  L2 : Constant  Value=0
  Mux : Mux  Inputs=6
  PS3_BT_Power : Constant  Value=0
  PS3_VSP_Speed : Constant  Value=0
  R2 : Constant  Value=0
  ScalingLX : Gain  Gain=1/32767
  ScalingLY : Gain  Gain=1/32767
  ScalingRY : Gain  Gain=1/32767
  Scaling_RX : Gain  Gain=1/32767
  DuelShock 3 signals : Outport
  PS3 BT Power : Outport  Port=2
  PS3 VSP Speed : Outport  Port=3
  wires:
  PS3_VSP_Speed/1 -> PS3 VSP Speed/1  "Voith Schnider Propeller Speed"
  PS3_BT_Power/1 -> PS3 BT Power/1  "Bow Thruster Power limit"
  Mux/1 -> DuelShock 3 signals/1
  AS_LX/1 -> ScalingLX/1  "x-position of left analog stick [-32767,32767]"
  ScalingLX/1 -> Mux/1  "x-position of left analog stick [-1,1]"
  AS_LY/1 -> ScalingLY/1  "y-position of left analog stick [-32767,32767]"
  ScalingLY/1 -> Mux/2  "y-position of left analog stick [-1,1]"
  AS_RX/1 -> Scaling_RX/1  "x-position of right analog stick  [-32767,32767]"
  Scaling_RX/1 -> Mux/3  "x-position of right analog stick  [-1,1]"
  ScalingRY/1 -> Mux/4  "y-position of right analog stick [-1,1]"
  AS_RY/1 -> ScalingRY/1  "y-position of right analog stick [-32767,32767]"
  L2/1 -> Mux/5  "L2 Button [-1,0]"
  R2/1 -> Mux/6  "R2 Button [0,1]"

== system CSE1_CV3_1Straight/Control Systems/Precision control ==
  note: The precision control is intended for getting accurate measurement of force generated from thrusters
  LabVIEW  BT power : Constant  Value=0
  LabVIEW VSP speed : Constant  Value=0
  LabVIEW u_{1..5} (5 alike) : Gain  ParameterDataType=fixdt(1, 16)  ParameterScaling=2^0  OutDataType=fixdt(1, 16)  OutScaling=2^0
  Mux2 : Mux  Inputs=7
  Subsystem : Subsystem
  u{1..5} (5 alike) : Constant  Value=0
  Thruster setting : Outport
  tau : Outport  Port=2
  wires:
  u1/1 -> LabVIEW u_1/1
  u2/1 -> LabVIEW u_2/1
  u3/1 -> LabVIEW u_3/1
  LabVIEW u_1/1 -> Mux2/1
  LabVIEW u_3/1 -> Mux2/3
  LabVIEW u_2/1 -> Mux2/2
  u4/1 -> LabVIEW u_4/1
  u5/1 -> LabVIEW u_5/1
  LabVIEW u_4/1 -> Mux2/4
  LabVIEW u_5/1 -> Mux2/5
  Mux2/1 -> Thruster setting/1, Subsystem/1(u_act)
  LabVIEW  BT power/1 -> Mux2/6
  LabVIEW VSP speed/1 -> Mux2/7
  Subsystem/1(tau) -> tau/1

== system CSE1_CV3_1Straight/Control Systems/Simple Control ==
  note: The control provides a more intuire control then manual thruster control
  PS3 Signals : Inport
  PS3 BT Power : Inport  Port=2
  PS3 VSP Speed : Inport  Port=3
  Demux1 : Demux  Outputs=6
  Demux2 : Demux  Outputs=5
  Joystick u_{1..5} (5 alike) : Gain  ParameterDataType=fixdt(1, 16)  ParameterScaling=2^0  OutDataType=fixdt(1, 16)  OutScaling=2^0
  Mux : Mux  Inputs=3
  Mux1 : Mux  Inputs=3
  Mux2 : Mux  Inputs=5
  Saturation : Saturate  UpperLimit=1.0  LowerLimit=-1.0
  Sum : Sum
  Sum1 : Sum
  Sum2 : Sum
  Thruster allocation : Subsystem
  tau_surge : Gain
  tau_sway : Gain
  tau_yaw : Gain
  Thruster setting : Outport
  tau : Outport  Port=2
  wires:
  PS3 Signals/1 -> Demux1/1
  Demux1/5 -> Sum/1
  Demux1/6 -> Sum/2
  Sum/1 -> tau_yaw/1
  Mux/1 -> Thruster allocation/1(tau), tau/1
  Mux1/1 -> Thruster setting/1
  PS3 BT Power/1 -> Mux1/2
  PS3 VSP Speed/1 -> Mux1/3
  Thruster allocation/1(u_act) -> Saturation/1
  Demux1/4 -> Sum1/2
  Demux1/2 -> Sum1/1
  Sum1/1 -> tau_surge/1
  Demux1/1 -> Sum2/1
  Demux1/3 -> Sum2/2
  Sum2/1 -> tau_sway/1
  Demux2/1 -> Joystick u_1/1
  Demux2/2 -> Joystick u_2/1
  Demux2/3 -> Joystick u_3/1
  Joystick u_1/1 -> Mux2/1
  Joystick u_3/1 -> Mux2/3
  Joystick u_2/1 -> Mux2/2
  Demux2/4 -> Joystick u_4/1
  Demux2/5 -> Joystick u_5/1
  Joystick u_4/1 -> Mux2/4
  Joystick u_5/1 -> Mux2/5
  Saturation/1 -> Demux2/1
  Mux2/1 -> Mux1/1
  tau_surge/1 -> Mux/1
  tau_sway/1 -> Mux/2
  tau_yaw/1 -> Mux/3

== system CSE1_CV3_1Straight/Guidance Systems/DP ==
  DP input : Inport
  Demux : Demux  Outputs=3
  Demux1 : Demux  Outputs=3
  Enable eta_d LPF : Constant  Value=0  OutDataType=fixdt(1, 16)  OutScaling=2^0
  Multiport Switch : MultiPortSwitch  Inputs=2  zeroidx=on  OutDataType=fixdt(1, 16)  OutScaling=2^0
  Mux : Mux  Inputs=3
  Mux1 : Mux  Inputs=3
  Terminator : Terminator
  Transfer Fcn : TransferFcn  Numerator=[0.1]  Denominator=[1 0.1]
  Transfer Fcn1 : TransferFcn  Numerator=[0.1]  Denominator=[1 0.1]
  Transfer Fcn2 : TransferFcn  Numerator=[0.1]  Denominator=[1 0.1]
  eta_d DP E : Gain  ParameterDataType=fixdt(1, 16)  ParameterScaling=2^0  OutDataType=fixdt(1, 16)  OutScaling=2^0
  eta_d DP N : Gain  ParameterDataType=fixdt(1, 16)  ParameterScaling=2^0  OutDataType=fixdt(1, 16)  OutScaling=2^0
  eta_d DP Psi : Gain  ParameterDataType=fixdt(1, 16)  ParameterScaling=2^0  OutDataType=fixdt(1, 16)  OutScaling=2^0
  eta_d Psi deg : Gain  Gain=180/pi  ParameterDataType=fixdt(1, 16)  ParameterScaling=2^0  OutDataType=fixdt(1, 16)  OutScaling=2^0
  DP eta_d : Outport
  wires:
  Enable eta_d LPF/1 -> Multiport Switch/1
  Mux1/1 -> Multiport Switch/3
  Demux/1 -> Transfer Fcn/1
  Transfer Fcn/1 -> Mux1/1
  Demux/2 -> Transfer Fcn1/1
  Transfer Fcn1/1 -> Mux1/2
  Demux/3 -> Transfer Fcn2/1
  Transfer Fcn2/1 -> Mux1/3
  DP input/1 -> Multiport Switch/2, Demux/1
  Multiport Switch/1 -> Demux1/1
  eta_d DP N/1 -> Mux/1
  eta_d DP E/1 -> Mux/2
  eta_d DP Psi/1 -> Mux/3
  Demux1/1 -> eta_d DP N/1
  Demux1/2 -> eta_d DP E/1
  Demux1/3 -> eta_d DP Psi/1, eta_d Psi deg/1
  Mux/1 -> DP eta_d/1
  eta_d Psi deg/1 -> Terminator/1

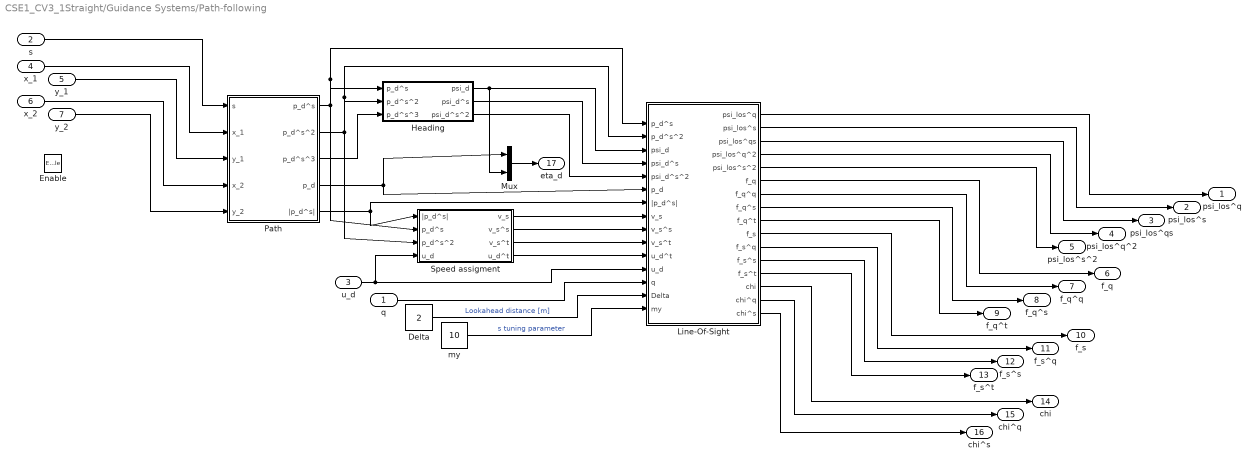
== system CSE1_CV3_1Straight/Guidance Systems/Path-following ==
  q : Inport
  s : Inport  Port=2
  u_d : Inport  Port=3
  x_1 : Inport  Port=4
  y_1 : Inport  Port=5
  x_2 : Inport  Port=6
  y_2 : Inport  Port=7
  Enable : EnablePort
  Delta : Constant  Value=2  OutDataType=fixdt(1, 16)  OutScaling=2^0
  Heading : Subsystem
  Line-Of-Sight : Subsystem
  Mux : Mux  Inputs=2
  Path : Subsystem
  Speed assigment : Subsystem
  my : Constant  Value=10  OutDataType=fixdt(1, 16)  OutScaling=2^0
  psi_los^q : Outport
  psi_los^s : Outport  Port=2
  psi_los^qs : Outport  Port=3
  psi_los^q^2 : Outport  Port=4
  psi_los^s^2 : Outport  Port=5
  f_q : Outport  Port=6
  "f_q^q " : Outport  Port=7
  f_q^s : Outport  Port=8
  f_q^t : Outport  Port=9
  f_s : Outport  Port=10
  f_s^q : Outport  Port=11
  f_s^s : Outport  Port=12
  f_s^t : Outport  Port=13
  chi : Outport  Port=14
  chi^q : Outport  Port=15
  chi^s : Outport  Port=16
  eta_d : Outport  Port=17
  wires:
  u_d/1 -> Line-Of-Sight/12(u_d), Speed assigment/4(u_d)
  Path/1(p_d^s) -> Speed assigment/2(p_d^s), Heading/1(p_d^s), Line-Of-Sight/1(p_d^s)
  x_2/1 -> Path/4(x_2)
  y_2/1 -> Path/5(y_2)
  x_1/1 -> Path/2(x_1)
  y_1/1 -> Path/3(y_1)
  s/1 -> Path/1(s)
  Heading/1(psi_d) -> Line-Of-Sight/3(psi_d), Mux/2
  Path/5(|p_d^s|) -> Line-Of-Sight/7(|p_d^s|), Speed assigment/1(|p_d^s|)
  Path/4(p_d) -> Line-Of-Sight/6(p_d), Mux/1
  Speed assigment/1(v_s) -> Line-Of-Sight/8(v_s)
  q/1 -> Line-Of-Sight/13(q)
  Path/2(p_d^s^2) -> Heading/2(p_d^s^2), Line-Of-Sight/2(p_d^s^2), Speed assigment/3(p_d^s^2)
  Heading/2(psi_d^s) -> Line-Of-Sight/4(psi_d^s)
  Path/3(p_d^s^3) -> Heading/3(p_d^s^3)
  Heading/3(psi_d^s^2) -> Line-Of-Sight/5(psi_d^s^2)
  Speed assigment/2(v_s^s) -> Line-Of-Sight/9(v_s^s)
  Line-Of-Sight/1(psi_los^q) -> psi_los^q/1
  Line-Of-Sight/2(psi_los^s) -> psi_los^s/1
  Line-Of-Sight/3(psi_los^qs) -> psi_los^qs/1
  Line-Of-Sight/4(psi_los^q^2) -> psi_los^q^2/1
  Line-Of-Sight/5(psi_los^s^2) -> psi_los^s^2/1
  Line-Of-Sight/6(f_q) -> f_q/1
  Line-Of-Sight/7("f_q^q ") -> "f_q^q "/1
  Line-Of-Sight/8(f_q^s) -> f_q^s/1
  Line-Of-Sight/9(f_q^t) -> f_q^t/1
  Line-Of-Sight/10(f_s) -> f_s/1
  Line-Of-Sight/11(f_s^q) -> f_s^q/1
  Line-Of-Sight/12(f_s^s) -> f_s^s/1
  Line-Of-Sight/13(f_s^t) -> f_s^t/1
  Line-Of-Sight/14(chi) -> chi/1
  Line-Of-Sight/15(chi^q) -> chi^q/1
  Line-Of-Sight/16(chi^s) -> chi^s/1
  Speed assigment/4(u_d^t) -> Line-Of-Sight/11(u_d^t)
  Speed assigment/3(v_s^t) -> Line-Of-Sight/10(v_s^t)
  Delta/1 -> Line-Of-Sight/14(Delta)  "Lookahead distance [m]"
  my/1 -> Line-Of-Sight/15(my)  "s tuning parameter"
  Mux/1 -> eta_d/1

== system CSE1_CV3_1Straight/HMI/DP Input ==
  Degrees to Radians : simulink_extras/Transformations/Degrees to Radians  SystemSampleTime=-1
  Mux : Mux  Inputs=3
  psi_d : Constant  Value=0
  x_d : Constant  Value=0
  y_d : Constant  Value=0
  DP input : Outport
  wires:
  x_d/1 -> Mux/1
  y_d/1 -> Mux/2
  Mux/1 -> DP input/1
  psi_d/1 -> Degrees to Radians/1
  Degrees to Radians/1 -> Mux/3

== system CSE1_CV3_1Straight/HMI/Path-following input ==
  Mux : Mux  Inputs=5
  u_d : Constant  Value=0.15  OutDataType=fixdt(1, 16)  OutScaling=2^0
  x_1 : Constant  Value=0  OutDataType=fixdt(1, 16)  OutScaling=2^0
  x_2 : Constant  Value=5.5  OutDataType=fixdt(1, 16)  OutScaling=2^0
  y_1 : Constant  Value=0  OutDataType=fixdt(1, 16)  OutScaling=2^0
  y_2 : Constant  Value=2  OutDataType=fixdt(1, 16)  OutScaling=2^0
  Path input : Outport
  wires:
  Mux/1 -> Path input/1
  u_d/1 -> Mux/1  "Desired speed [m/s]"
  x_1/1 -> Mux/2  "x-coord. reference point straight path [m]"
  y_1/1 -> Mux/3  "y-coord, reference point straight path [m]"
  x_2/1 -> Mux/4  "x-coord, direction point straigth path [m]"
  y_2/1 -> Mux/5  "y-coord, direction point straigth path [m]"

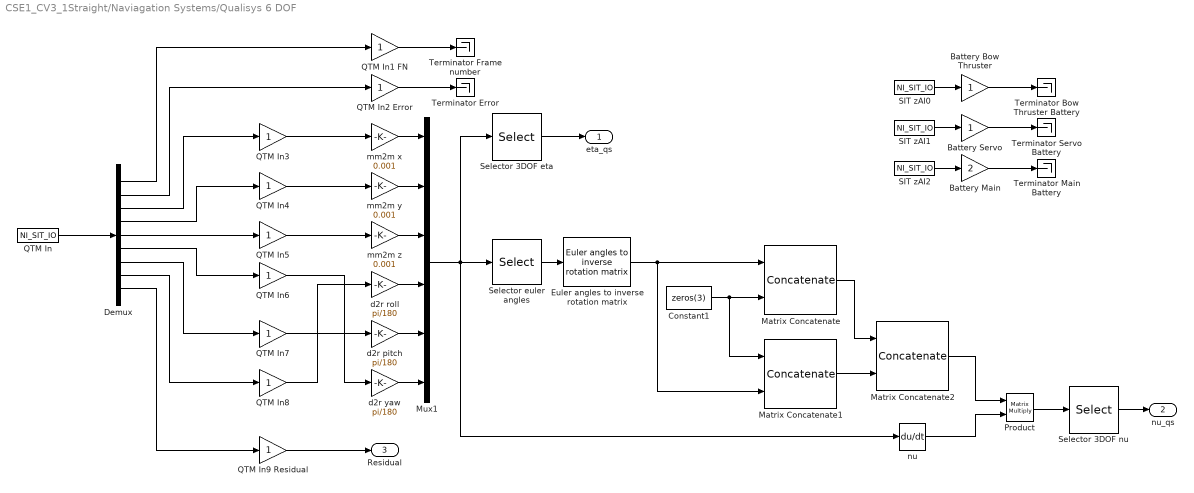
== system CSE1_CV3_1Straight/Naviagation Systems/Qualisys 6 DOF ==
  Battery Bow Thruster : Gain  ParameterDataType=fixdt(1, 16)  ParameterScaling=2^0  OutDataType=fixdt(1, 16)  OutScaling=2^0
  Battery Main : Gain  Gain=2  ParameterDataType=fixdt(1, 16)  ParameterScaling=2^0  OutDataType=fixdt(1, 16)  OutScaling=2^0
  Battery Servo : Gain  ParameterDataType=fixdt(1, 16)  ParameterScaling=2^0  OutDataType=fixdt(1, 16)  OutScaling=2^0
  Constant1 : Constant  Value=zeros(3)
  Demux : Demux  Outputs=9
  Euler angles to inverse rotation matrix : marine_gnc/Models/ Kinematics/Euler angles to inverse rotation matrix  SystemSampleTime=-1
  Matrix Concatenate : Concatenate  Mode=Multidimensional array
  Matrix Concatenate1 : Concatenate  Mode=Multidimensional array
  Matrix Concatenate2 : Concatenate  Mode=Multidimensional array  ConcatenateDimension=2
  Mux1 : Mux  Inputs=6
  Product : Product  Multiplication=Matrix(*)  RndMeth=Zero
  QTM In : S-Function  Priority=1  FunctionName=NI_SIT_IO  Parameters=width dtype portnum stime stype btype  EnableBusSupport=off  mask(SIT Inport){portnum=1, width=9, stime=-1, dtype=auto, stype=auto, btype=1}
      mask prompts: portnum "Port number:"; width "Port dimensions (-1 for dynamically sized):"; stime "Sample time (-1 for inherited):"; dtype "Data type:"; stype "Signal type:"; btype "Block type:"
      mask help: Use this inport on any level of nested subsystems to allow the LabVIEW Simulation Interface Toolkit to map hardware to it.
      mask init:
      | NI_SIT_IO_init;
      settings: CopyFcn=NI_SIT_IO_callbacks(1);  DeleteFcn=NI_SIT_IO_callbacks(2);
      mask StyleString: edit,edit,edit,popup(auto|double|single|int8|uint8|int16|uint16|int32|uint32|boolean),popup(auto|real|complex),edit
      mask CallbackString: NI_SIT_IO_callbacks(3);|||NI_SIT_IO_callbacks(4);||
      mask TabNameString: Parameters,Parameters,Parameters,Parameters,Parameters,Parameters
      mask Display:
      | patch([-x x], [-y y], [.90980 .81960 .32156]);
      | plot([0 -x x 0], [rad -y y rad]);
      | fprintf('SIT%d', portnum);
  QTM In1 FN : Gain  ParameterDataType=fixdt(1, 16)  ParameterScaling=2^0  OutDataType=fixdt(1, 16)  OutScaling=2^0
  QTM In2 Error : Gain  ParameterDataType=fixdt(1, 16)  ParameterScaling=2^0  OutDataType=fixdt(1, 16)  OutScaling=2^0
  QTM In{3..8} (6 alike) : Gain  ParameterDataType=fixdt(1, 16)  ParameterScaling=2^0  OutDataType=fixdt(1, 16)  OutScaling=2^0
  QTM In9 Residual : Gain  ParameterDataType=fixdt(1, 16)  ParameterScaling=2^0  OutDataType=fixdt(1, 16)  OutScaling=2^0
  SIT zAI0 : S-Function  Priority=4  FunctionName=NI_SIT_IO  Parameters=width dtype portnum stime stype btype  EnableBusSupport=off  mask(SIT Inport){portnum=4, width=-1, stime=-1, dtype=auto, stype=auto, btype=1}
      mask prompts: portnum "Port number:"; width "Port dimensions (-1 for dynamically sized):"; stime "Sample time (-1 for inherited):"; dtype "Data type:"; stype "Signal type:"; btype "Block type:"
      mask help: Use this inport on any level of nested subsystems to allow the LabVIEW Simulation Interface Toolkit to map hardware to it.
      mask init:
      | NI_SIT_IO_init;
      settings: CopyFcn=NI_SIT_IO_callbacks(1);  DeleteFcn=NI_SIT_IO_callbacks(2);
      mask StyleString: edit,edit,edit,popup(auto|double|single|int8|uint8|int16|uint16|int32|uint32|boolean),popup(auto|real|complex),edit
      mask CallbackString: NI_SIT_IO_callbacks(3);|||NI_SIT_IO_callbacks(4);||
      mask TabNameString: Parameters,Parameters,Parameters,Parameters,Parameters,Parameters
      mask Display:
      | patch([-x x], [-y y], [.90980 .81960 .32156]);
      | plot([0 -x x 0], [rad -y y rad]);
      | fprintf('SIT%d', portnum);
  SIT zAI1 : S-Function  Priority=2  FunctionName=NI_SIT_IO  Parameters=width dtype portnum stime stype btype  EnableBusSupport=off  mask(SIT Inport){portnum=2, width=-1, stime=-1, dtype=auto, stype=auto, btype=1}
      mask prompts: portnum "Port number:"; width "Port dimensions (-1 for dynamically sized):"; stime "Sample time (-1 for inherited):"; dtype "Data type:"; stype "Signal type:"; btype "Block type:"
      mask help: Use this inport on any level of nested subsystems to allow the LabVIEW Simulation Interface Toolkit to map hardware to it.
      mask init:
      | NI_SIT_IO_init;
      settings: CopyFcn=NI_SIT_IO_callbacks(1);  DeleteFcn=NI_SIT_IO_callbacks(2);
      mask StyleString: edit,edit,edit,popup(auto|double|single|int8|uint8|int16|uint16|int32|uint32|boolean),popup(auto|real|complex),edit
      mask CallbackString: NI_SIT_IO_callbacks(3);|||NI_SIT_IO_callbacks(4);||
      mask TabNameString: Parameters,Parameters,Parameters,Parameters,Parameters,Parameters
      mask Display:
      | patch([-x x], [-y y], [.90980 .81960 .32156]);
      | plot([0 -x x 0], [rad -y y rad]);
      | fprintf('SIT%d', portnum);
  SIT zAI2 : S-Function  Priority=3  FunctionName=NI_SIT_IO  Parameters=width dtype portnum stime stype btype  EnableBusSupport=off  mask(SIT Inport){portnum=3, width=-1, stime=-1, dtype=auto, stype=auto, btype=1}
      mask prompts: portnum "Port number:"; width "Port dimensions (-1 for dynamically sized):"; stime "Sample time (-1 for inherited):"; dtype "Data type:"; stype "Signal type:"; btype "Block type:"
      mask help: Use this inport on any level of nested subsystems to allow the LabVIEW Simulation Interface Toolkit to map hardware to it.
      mask init:
      | NI_SIT_IO_init;
      settings: CopyFcn=NI_SIT_IO_callbacks(1);  DeleteFcn=NI_SIT_IO_callbacks(2);
      mask StyleString: edit,edit,edit,popup(auto|double|single|int8|uint8|int16|uint16|int32|uint32|boolean),popup(auto|real|complex),edit
      mask CallbackString: NI_SIT_IO_callbacks(3);|||NI_SIT_IO_callbacks(4);||
      mask TabNameString: Parameters,Parameters,Parameters,Parameters,Parameters,Parameters
      mask Display:
      | patch([-x x], [-y y], [.90980 .81960 .32156]);
      | plot([0 -x x 0], [rad -y y rad]);
      | fprintf('SIT%d', portnum);
  Selector 3DOF eta : Selector  InputPortWidth=6  IndexOptions=Index vector (dialog)  Indices=[1 2 6]  OutputSizes=1
  Selector 3DOF nu : Selector  InputPortWidth=6  IndexOptions=Index vector (dialog)  Indices=[1 2 6]  OutputSizes=1
  Selector euler angles : Selector  InputPortWidth=6  IndexOptions=Index vector (dialog)  Indices=[4 5 6]  OutputSizes=1
  Terminator Bow Thruster Battery : Terminator
  Terminator Error : Terminator
  Terminator Frame number : Terminator
  Terminator Main Battery : Terminator
  Terminator Servo Battery : Terminator
  d2r pitch : Gain  Gain=pi/180  ParameterDataType=fixdt(1, 16)  ParameterScaling=2^0  OutDataType=fixdt(1, 16)  OutScaling=2^0
  d2r roll : Gain  Gain=pi/180  ParameterDataType=fixdt(1, 16)  ParameterScaling=2^0  OutDataType=fixdt(1, 16)  OutScaling=2^0
  d2r yaw : Gain  Gain=pi/180  ParameterDataType=fixdt(1, 16)  ParameterScaling=2^0  OutDataType=fixdt(1, 16)  OutScaling=2^0
  mm2m x : Gain  Gain=0.001
  mm2m y : Gain  Gain=0.001
  mm2m z : Gain  Gain=0.001
  nu : Derivative
  eta_qs : Outport
  nu_qs : Outport  Port=2
  Residual : Outport  Port=3
  wires:
  Mux1/1 -> Selector euler angles/1, Selector 3DOF eta/1, nu/1
  Selector 3DOF eta/1 -> eta_qs/1
  Euler angles to inverse rotation matrix/1 -> Matrix Concatenate/1, Matrix Concatenate1/2
  Matrix Concatenate/1 -> Matrix Concatenate2/1
  Matrix Concatenate1/1 -> Matrix Concatenate2/2
  Matrix Concatenate2/1 -> Product/1
  nu/1 -> Product/2
  Constant1/1 -> Matrix Concatenate/2, Matrix Concatenate1/1
  mm2m z/1 -> Mux1/3
  mm2m y/1 -> Mux1/2
  mm2m x/1 -> Mux1/1
  d2r yaw/1 -> Mux1/6
  d2r pitch/1 -> Mux1/5
  d2r roll/1 -> Mux1/4
  Selector euler angles/1 -> Euler angles to inverse rotation matrix/1
  Product/1 -> Selector 3DOF nu/1
  Selector 3DOF nu/1 -> nu_qs/1
  QTM In1 FN/1 -> Terminator Frame number/1
  QTM In/1 -> Demux/1
  Demux/1 -> QTM In1 FN/1
  Demux/2 -> QTM In2 Error/1
  Demux/3 -> QTM In3/1
  Demux/4 -> QTM In4/1
  Demux/5 -> QTM In5/1
  Demux/6 -> QTM In6/1
  Demux/7 -> QTM In7/1
  Demux/8 -> QTM In8/1
  Demux/9 -> QTM In9 Residual/1
  QTM In3/1 -> mm2m x/1
  QTM In4/1 -> mm2m y/1
  QTM In5/1 -> mm2m z/1
  QTM In7/1 -> d2r pitch/1
  QTM In6/1 -> d2r yaw/1
  QTM In8/1 -> d2r roll/1
  QTM In2 Error/1 -> Terminator Error/1
  QTM In9 Residual/1 -> Residual/1
  SIT zAI0/1 -> Battery Bow Thruster/1
  SIT zAI1/1 -> Battery Servo/1
  SIT zAI2/1 -> Battery Main/1
  Battery Bow Thruster/1 -> Terminator Bow Thruster Battery/1
  Battery Servo/1 -> Terminator Servo Battery/1
  Battery Main/1 -> Terminator Main Battery/1
